simulink model "simulate_P_controller"  (R2024b)
settings: Solver=ode4  StartTime=0.0  StopTime=Tfin  FixedStep=Tc  RelTol=1e-3
undefined symbols (not defined in the file): Kp_1
settings Model: Creator=martinhaugen  LastModifiedBy=martinhaugen

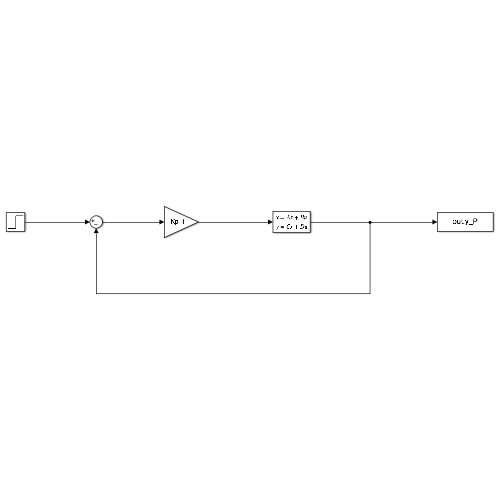
[thumbnail: Simulink's stored preview of the top-level diagram]
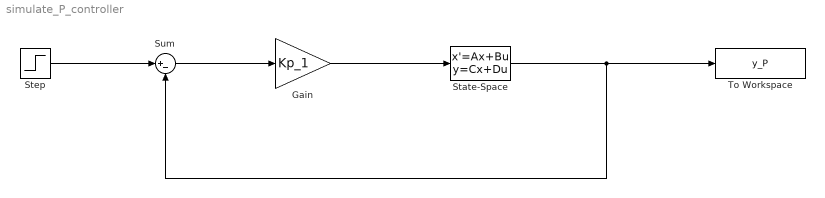
== system simulate_P_controller ==
  Gain : Gain  Gain=Kp_1
  State-Space : StateSpace  InitialCondition=0
  Step : Step  Time=0  SampleTime=0
  Sum : Sum  Inputs=|+-
  To Workspace : ToWorkspace  VariableName=y_P  SampleTime=-1
  wires:
  Step/1 -> Sum/1
  Sum/1 -> Gain/1
  Gain/1 -> State-Space/1
  State-Space/1 -> To Workspace/1, Sum/2
